simulink model "FullDecoder3"  (R2020b)
settings: Solver=FixedStepDiscrete  StartTime=0.0  StopTime=60  FixedStep=1.0000e-04  RelTol=1e-3
settings Model: Creator=micha  LastModifiedBy=micha
settings DataIOCC: ReturnWorkspaceOutputs=off

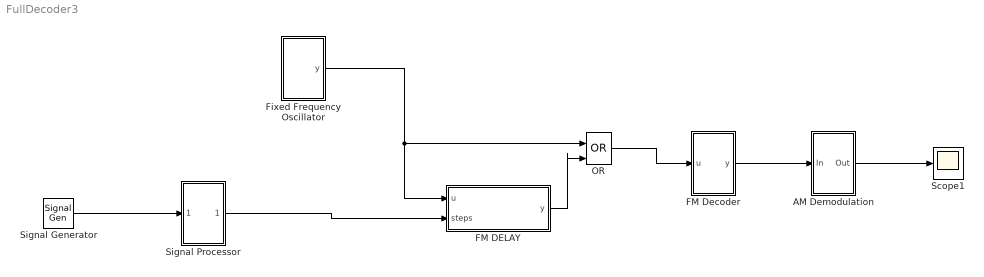
== system FullDecoder3 ==
  AM Demodulation : Subsystem
  FM DELAY : MATLAB Function  TreatAsAtomicUnit=on
  FM Decoder : Subsystem
  Fixed Frequency Oscillator : Subsystem
  OR : Logic  Operator=OR  IconShape=distinctive  AllPortsSameDT=off  OutDataTypeStr=boolean
  Scope1 : Scope
  Signal Generator : SignalGenerator
  Signal Processor : Subsystem
  wires:
  AM Demodulation/1(Out) -> Scope1/1
  FM DELAY/1(y) -> OR/2
  Fixed Frequency Oscillator/1(y) -> FM DELAY/1(u), OR/1
  OR/1 -> FM Decoder/1(u)
  FM Decoder/1(y) -> AM Demodulation/1(In)
  Signal Processor/1(Out1) -> FM DELAY/2(steps)
  Signal Generator/1 -> Signal Processor/1(Input)

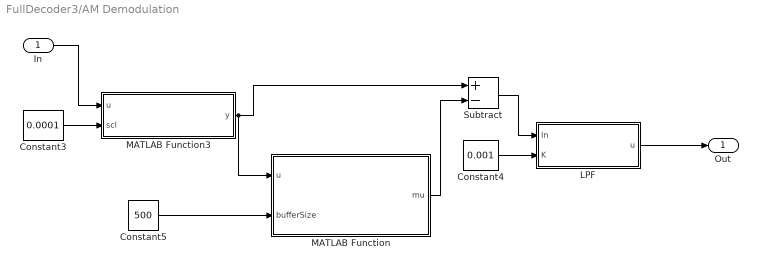
== system FullDecoder3/AM Demodulation ==
  In : Inport
  Constant3 : Constant  Value=0.0001
  Constant4 : Constant  Value=0.001
  Constant5 : Constant  Value=500  OutDataTypeStr=int16
  LPF : Subsystem
  MATLAB Function : MATLAB Function  TreatAsAtomicUnit=on
  MATLAB Function3 : MATLAB Function  TreatAsAtomicUnit=on
  Subtract : Sum  Inputs=+-
  Out : Outport
  wires:
  MATLAB Function3/1(y) -> Subtract/1, MATLAB Function/1(u)
  Constant5/1 -> MATLAB Function/2(bufferSize)
  Constant3/1 -> MATLAB Function3/2(scl)
  MATLAB Function/1(mu) -> Subtract/2
  Constant4/1 -> LPF/2(K)
  In/1 -> MATLAB Function3/1(u)
  Subtract/1 -> LPF/1(In)
  LPF/1(u) -> Out/1

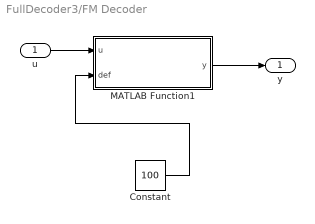
== system FullDecoder3/FM Decoder ==
  u : Inport
  Constant : Constant  Value=100
  MATLAB Function1 : MATLAB Function  TreatAsAtomicUnit=on
  y : Outport
  wires:
  Constant/1 -> MATLAB Function1/2(def)
  u/1 -> MATLAB Function1/1(u)
  MATLAB Function1/1(y) -> y/1

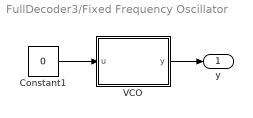
== system FullDecoder3/Fixed Frequency Oscillator ==
  Constant1 : Constant  Value=0
  VCO : MATLAB Function  TreatAsAtomicUnit=on
  y : Outport
  wires:
  Constant1/1 -> VCO/1(u)
  VCO/1(y) -> y/1

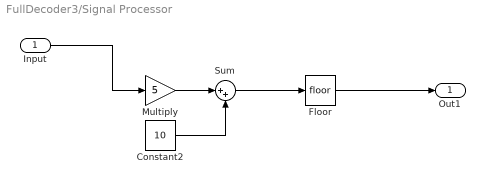
== system FullDecoder3/Signal Processor ==
  Input : Inport
  Constant2 : Constant  Value=10
  Floor : Rounding
  Multiply : Gain  Gain=5
  Sum : Sum  Inputs=|++
  Out1 : Outport
  wires:
  Sum/1 -> Floor/1
  Input/1 -> Multiply/1
  Floor/1 -> Out1/1
  Constant2/1 -> Sum/2
  Multiply/1 -> Sum/1

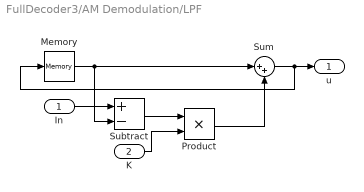
== system FullDecoder3/AM Demodulation/LPF ==
  In : Inport
  K : Inport  Port=2
  Memory : Memory
  Product : Product
  Subtract : Sum  Inputs=+-
  Sum : Sum  Inputs=|++
  u : Outport
  wires:
  Product/1 -> Sum/2
  Subtract/1 -> Product/1
  In/1 -> Subtract/1
  K/1 -> Product/2
  Memory/1 -> Subtract/2, Sum/1
  Sum/1 -> u/1, Memory/1

== matlab function FullDecoder3/Fixed Frequency Oscillator/VCO ==
  data: u input; y output
function y = fmEncoder(u)
timeStep=1e-4;
defaultWait=0.01;
deltaWait=0.005;
persistent timer

if isempty(timer)
    timer=0;
    
end
timer=timer-timeStep;
if timer<0
    y=1;
    timer=defaultWait-u*deltaWait;
else
   y=0; 
end

end

== matlab function FullDecoder3/AM Demodulation/MATLAB Function ==
  data: u input; mu output; bufferSize input

function mu =BufferMean(u,bufferSize)
    persistent buffer
    if (isempty(buffer))
        buffer=zeros(1,bufferSize);
    end
    for i=1:bufferSize-1
        buffer(i)=buffer(i+1);
    end
    buffer(bufferSize)=u;
    
    mu=mean(buffer);
end

== matlab function FullDecoder3/AM Demodulation/MATLAB Function3 ==
  data: u input; y output; scl input
function y = EnvelopeDetector(u,scl)
persistent state
if isempty(state)
state=0;
end 


y = state+scl*(u-state);
state=y;

== matlab function FullDecoder3/FM DELAY ==
  data: u input; y output; steps input
function y = delay(u,steps)
persistent buffer
if(isempty(buffer))
   buffer=zeros(1,5000); 
end
if steps>0
y = buffer(1);
for i=1:steps-1
   buffer(i)=buffer(i+1); 
end
buffer(steps)=u;
else
    y=u;
end

== matlab function FullDecoder3/FM Decoder/MATLAB Function1 ==
  data: u input; y output; def input
function y = fmDecoder(u,def)
persistent counter;
persistent state;
if isempty(counter)
   counter=0;
end
if(isempty(state))
   state=0; 
end
y=state;
if u==0
    
   counter=counter+1;

end

if u==1
    y=def-counter;
    state=y;
   counter=0;
  
end




end
